simulink model "gm_hybrid_lht"  (R2019b)
settings: Solver=FixedStepDiscrete  StartTime=0.0  StopTime=inf  FixedStep=1/120e6  RelTol=1e-3
undefined symbols (not defined in the file or in its folder): bt, height, nTheta, width
libraries: hdlsllib x672, simulink x614, hdlmdlgenlib x7, dspsrcs4 x1
(part 10 of 18)

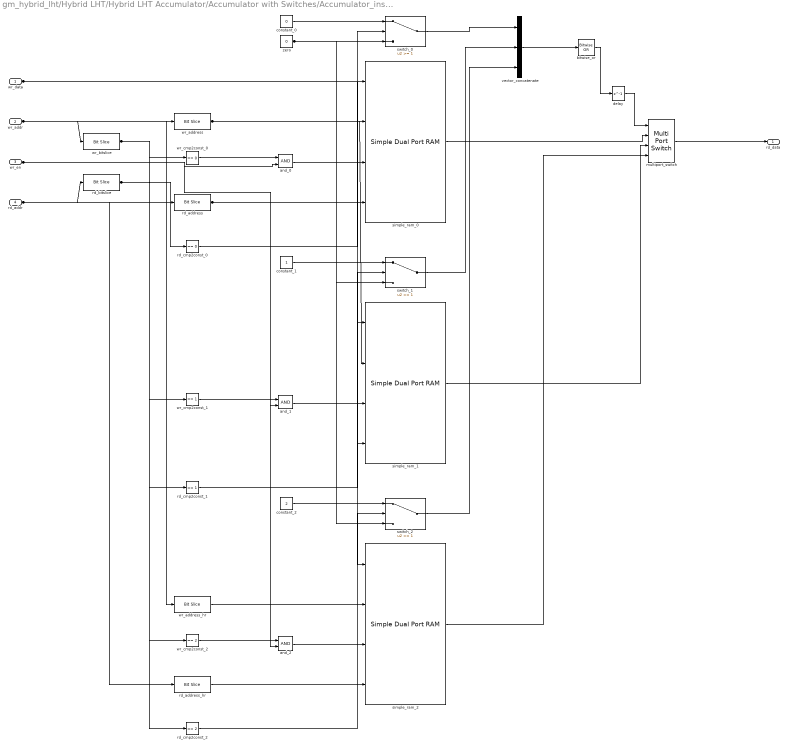
== system gm_hybrid_lht/Hybrid LHT/Hybrid LHT Accumulator/Accumulator with Switches/Accumulator_instance11/Block RAM/Simple Dual Port RAM Generator ==
  wr_data : Inport  OutDataTypeStr=fixdt(0, 36, 0)  PortDimensions=1  SampleTime=8.33333333333333e-09
  wr_addr : Inport  Port=2  OutDataTypeStr=fixdt(0, 12, 0)  PortDimensions=1  SampleTime=8.33333333333333e-09
  wr_en : Inport  Port=3  OutDataTypeStr=boolean  PortDimensions=1  SampleTime=8.33333333333333e-09
  rd_addr : Inport  Port=4  OutDataTypeStr=fixdt(0, 12, 0)  PortDimensions=1  SampleTime=8.33333333333333e-09
  and_0 : Logic  AllPortsSameDT=off  OutDataTypeStr=boolean
  and_1 : Logic  AllPortsSameDT=off  OutDataTypeStr=boolean
  and_2 : Logic  AllPortsSameDT=off  OutDataTypeStr=boolean
  bitwise_or : simulink/Logic and Bit Operations/Bitwise Operator  logicop=OR  UseBitMask=off  BitMask=bin2dec('11011001')  BitMaskRealWorld=Stored Integer
  constant_0 : Constant  Value=0  OutDataTypeStr=fixdt(0, 3, 0)  SampleTime=-1
  constant_1 : Constant  OutDataTypeStr=fixdt(0, 3, 0)  SampleTime=-1
  constant_2 : Constant  Value=2  OutDataTypeStr=fixdt(0, 3, 0)  SampleTime=-1
  delay : Delay  DelayLength=1
  multiport_switch : MultiPortSwitch  DataPortOrder=Zero-based contiguous  zeroidx=on
  rd_address : hdlsllib/Logic and Bit Operations/Bit Slice  lidx=9  ridx=0
      settings: SourceProductName=Simulink  SourceProductBaseCode=SL
  rd_address_hr : hdlsllib/Logic and Bit Operations/Bit Slice  lidx=8  ridx=0
      settings: SourceProductName=Simulink  SourceProductBaseCode=SL
  rd_bitslice : hdlsllib/Logic and Bit Operations/Bit Slice  lidx=11  ridx=10
      settings: SourceProductName=Simulink  SourceProductBaseCode=SL
  rd_cmp2const_0 : simulink/Logic and Bit Operations/Compare To Constant  relop===  const=0  OutDataTypeStr=boolean
  rd_cmp2const_1 : simulink/Logic and Bit Operations/Compare To Constant  relop===  const=1  OutDataTypeStr=boolean
  rd_cmp2const_2 : simulink/Logic and Bit Operations/Compare To Constant  relop===  const=2  OutDataTypeStr=boolean
  simple_ram_0 : hdlsllib/HDL RAMs/Simple Dual Port RAM  ram_size=10
      settings: SourceProductName=Simulink  SourceProductBaseCode=SL
  simple_ram_1 : hdlsllib/HDL RAMs/Simple Dual Port RAM  ram_size=10
      settings: SourceProductName=Simulink  SourceProductBaseCode=SL
  simple_ram_2 : hdlsllib/HDL RAMs/Simple Dual Port RAM  ram_size=9
      settings: SourceProductName=Simulink  SourceProductBaseCode=SL
  switch_0 : Switch  Threshold=1
  switch_1 : Switch  Threshold=1
  switch_2 : Switch  Threshold=1
  vector_concatenate : Concatenate  NumInputs=3
  wr_address : hdlsllib/Logic and Bit Operations/Bit Slice  lidx=9  ridx=0
      settings: SourceProductName=Simulink  SourceProductBaseCode=SL
  wr_address_hr : hdlsllib/Logic and Bit Operations/Bit Slice  lidx=8  ridx=0
      settings: SourceProductName=Simulink  SourceProductBaseCode=SL
  wr_bitslice : hdlsllib/Logic and Bit Operations/Bit Slice  lidx=11  ridx=10
      settings: SourceProductName=Simulink  SourceProductBaseCode=SL
  wr_cmp2const_0 : simulink/Logic and Bit Operations/Compare To Constant  relop===  const=0  OutDataTypeStr=boolean
  wr_cmp2const_1 : simulink/Logic and Bit Operations/Compare To Constant  relop===  const=1  OutDataTypeStr=boolean
  wr_cmp2const_2 : simulink/Logic and Bit Operations/Compare To Constant  relop===  const=2  OutDataTypeStr=boolean
  zero : Constant  Value=0  OutDataTypeStr=fixdt(0, 3, 0)  SampleTime=-1
  rd_data : Outport
  wires:
  rd_addr/1 -> rd_bitslice/1, rd_address_hr/1, rd_address/1
  wr_en/1 -> and_2/2, and_1/2, and_0/2
  wr_addr/1 -> wr_bitslice/1, wr_address_hr/1, wr_address/1
  wr_data/1 -> simple_ram_0/1, simple_ram_1/1, simple_ram_2/1
  and_0/1 -> simple_ram_0/3
  and_1/1 -> simple_ram_1/3
  and_2/1 -> simple_ram_2/3
  bitwise_or/1 -> delay/1
  constant_0/1 -> switch_0/1
  constant_1/1 -> switch_1/1
  constant_2/1 -> switch_2/1
  delay/1 -> multiport_switch/1
  multiport_switch/1 -> rd_data/1
  rd_address/1 -> simple_ram_0/4, simple_ram_1/4
  rd_address_hr/1 -> simple_ram_2/4
  rd_bitslice/1 -> rd_cmp2const_2/1, rd_cmp2const_1/1, rd_cmp2const_0/1
  rd_cmp2const_0/1 -> switch_0/2
  rd_cmp2const_1/1 -> switch_1/2
  rd_cmp2const_2/1 -> switch_2/2
  simple_ram_0/1 -> multiport_switch/2
  simple_ram_1/1 -> multiport_switch/3
  simple_ram_2/1 -> multiport_switch/4
  switch_0/1 -> vector_concatenate/1
  switch_1/1 -> vector_concatenate/2
  switch_2/1 -> vector_concatenate/3
  vector_concatenate/1 -> bitwise_or/1
  wr_address/1 -> simple_ram_0/2, simple_ram_1/2
  wr_address_hr/1 -> simple_ram_2/2
  wr_bitslice/1 -> wr_cmp2const_2/1, wr_cmp2const_1/1, wr_cmp2const_0/1
  wr_cmp2const_0/1 -> and_0/1
  wr_cmp2const_1/1 -> and_1/1
  wr_cmp2const_2/1 -> and_2/1
  zero/1 -> switch_2/3, switch_1/3, switch_0/3

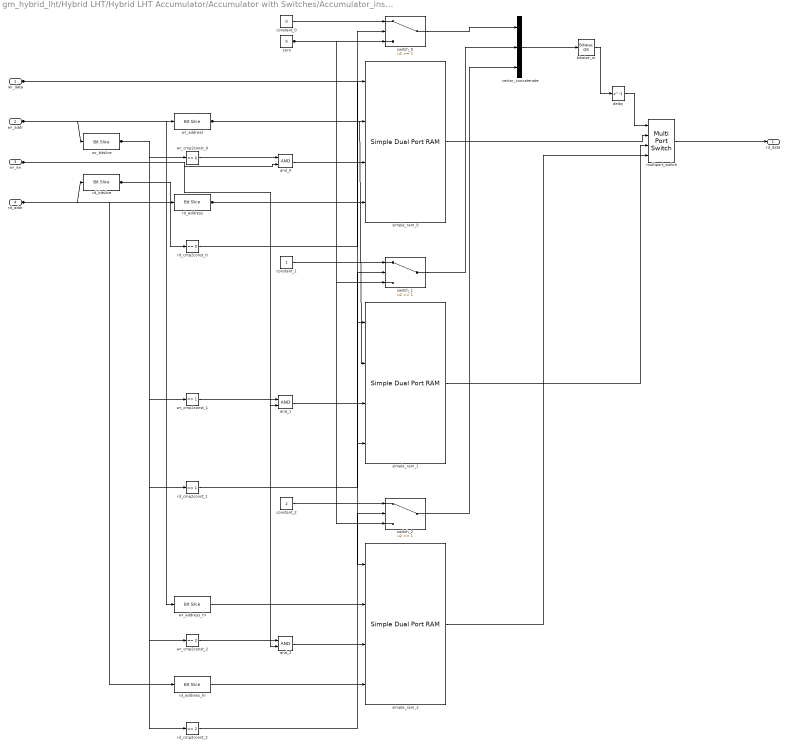
== system gm_hybrid_lht/Hybrid LHT/Hybrid LHT Accumulator/Accumulator with Switches/Accumulator_instance12/Block RAM/Simple Dual Port RAM Generator ==
  wr_data : Inport  OutDataTypeStr=fixdt(0, 36, 0)  PortDimensions=1  SampleTime=8.33333333333333e-09
  wr_addr : Inport  Port=2  OutDataTypeStr=fixdt(0, 12, 0)  PortDimensions=1  SampleTime=8.33333333333333e-09
  wr_en : Inport  Port=3  OutDataTypeStr=boolean  PortDimensions=1  SampleTime=8.33333333333333e-09
  rd_addr : Inport  Port=4  OutDataTypeStr=fixdt(0, 12, 0)  PortDimensions=1  SampleTime=8.33333333333333e-09
  and_0 : Logic  AllPortsSameDT=off  OutDataTypeStr=boolean
  and_1 : Logic  AllPortsSameDT=off  OutDataTypeStr=boolean
  and_2 : Logic  AllPortsSameDT=off  OutDataTypeStr=boolean
  bitwise_or : simulink/Logic and Bit Operations/Bitwise Operator  logicop=OR  UseBitMask=off  BitMask=bin2dec('11011001')  BitMaskRealWorld=Stored Integer
  constant_0 : Constant  Value=0  OutDataTypeStr=fixdt(0, 3, 0)  SampleTime=-1
  constant_1 : Constant  OutDataTypeStr=fixdt(0, 3, 0)  SampleTime=-1
  constant_2 : Constant  Value=2  OutDataTypeStr=fixdt(0, 3, 0)  SampleTime=-1
  delay : Delay  DelayLength=1
  multiport_switch : MultiPortSwitch  DataPortOrder=Zero-based contiguous  zeroidx=on
  rd_address : hdlsllib/Logic and Bit Operations/Bit Slice  lidx=9  ridx=0
      settings: SourceProductName=Simulink  SourceProductBaseCode=SL
  rd_address_hr : hdlsllib/Logic and Bit Operations/Bit Slice  lidx=8  ridx=0
      settings: SourceProductName=Simulink  SourceProductBaseCode=SL
  rd_bitslice : hdlsllib/Logic and Bit Operations/Bit Slice  lidx=11  ridx=10
      settings: SourceProductName=Simulink  SourceProductBaseCode=SL
  rd_cmp2const_0 : simulink/Logic and Bit Operations/Compare To Constant  relop===  const=0  OutDataTypeStr=boolean
  rd_cmp2const_1 : simulink/Logic and Bit Operations/Compare To Constant  relop===  const=1  OutDataTypeStr=boolean
  rd_cmp2const_2 : simulink/Logic and Bit Operations/Compare To Constant  relop===  const=2  OutDataTypeStr=boolean
  simple_ram_0 : hdlsllib/HDL RAMs/Simple Dual Port RAM  ram_size=10
      settings: SourceProductName=Simulink  SourceProductBaseCode=SL
  simple_ram_1 : hdlsllib/HDL RAMs/Simple Dual Port RAM  ram_size=10
      settings: SourceProductName=Simulink  SourceProductBaseCode=SL
  simple_ram_2 : hdlsllib/HDL RAMs/Simple Dual Port RAM  ram_size=9
      settings: SourceProductName=Simulink  SourceProductBaseCode=SL
  switch_0 : Switch  Threshold=1
  switch_1 : Switch  Threshold=1
  switch_2 : Switch  Threshold=1
  vector_concatenate : Concatenate  NumInputs=3
  wr_address : hdlsllib/Logic and Bit Operations/Bit Slice  lidx=9  ridx=0
      settings: SourceProductName=Simulink  SourceProductBaseCode=SL
  wr_address_hr : hdlsllib/Logic and Bit Operations/Bit Slice  lidx=8  ridx=0
      settings: SourceProductName=Simulink  SourceProductBaseCode=SL
  wr_bitslice : hdlsllib/Logic and Bit Operations/Bit Slice  lidx=11  ridx=10
      settings: SourceProductName=Simulink  SourceProductBaseCode=SL
  wr_cmp2const_0 : simulink/Logic and Bit Operations/Compare To Constant  relop===  const=0  OutDataTypeStr=boolean
  wr_cmp2const_1 : simulink/Logic and Bit Operations/Compare To Constant  relop===  const=1  OutDataTypeStr=boolean
  wr_cmp2const_2 : simulink/Logic and Bit Operations/Compare To Constant  relop===  const=2  OutDataTypeStr=boolean
  zero : Constant  Value=0  OutDataTypeStr=fixdt(0, 3, 0)  SampleTime=-1
  rd_data : Outport
  wires:
  rd_addr/1 -> rd_bitslice/1, rd_address_hr/1, rd_address/1
  wr_en/1 -> and_2/2, and_1/2, and_0/2
  wr_addr/1 -> wr_bitslice/1, wr_address_hr/1, wr_address/1
  wr_data/1 -> simple_ram_0/1, simple_ram_1/1, simple_ram_2/1
  and_0/1 -> simple_ram_0/3
  and_1/1 -> simple_ram_1/3
  and_2/1 -> simple_ram_2/3
  bitwise_or/1 -> delay/1
  constant_0/1 -> switch_0/1
  constant_1/1 -> switch_1/1
  constant_2/1 -> switch_2/1
  delay/1 -> multiport_switch/1
  multiport_switch/1 -> rd_data/1
  rd_address/1 -> simple_ram_0/4, simple_ram_1/4
  rd_address_hr/1 -> simple_ram_2/4
  rd_bitslice/1 -> rd_cmp2const_2/1, rd_cmp2const_1/1, rd_cmp2const_0/1
  rd_cmp2const_0/1 -> switch_0/2
  rd_cmp2const_1/1 -> switch_1/2
  rd_cmp2const_2/1 -> switch_2/2
  simple_ram_0/1 -> multiport_switch/2
  simple_ram_1/1 -> multiport_switch/3
  simple_ram_2/1 -> multiport_switch/4
  switch_0/1 -> vector_concatenate/1
  switch_1/1 -> vector_concatenate/2
  switch_2/1 -> vector_concatenate/3
  vector_concatenate/1 -> bitwise_or/1
  wr_address/1 -> simple_ram_0/2, simple_ram_1/2
  wr_address_hr/1 -> simple_ram_2/2
  wr_bitslice/1 -> wr_cmp2const_2/1, wr_cmp2const_1/1, wr_cmp2const_0/1
  wr_cmp2const_0/1 -> and_0/1
  wr_cmp2const_1/1 -> and_1/1
  wr_cmp2const_2/1 -> and_2/1
  zero/1 -> switch_2/3, switch_1/3, switch_0/3

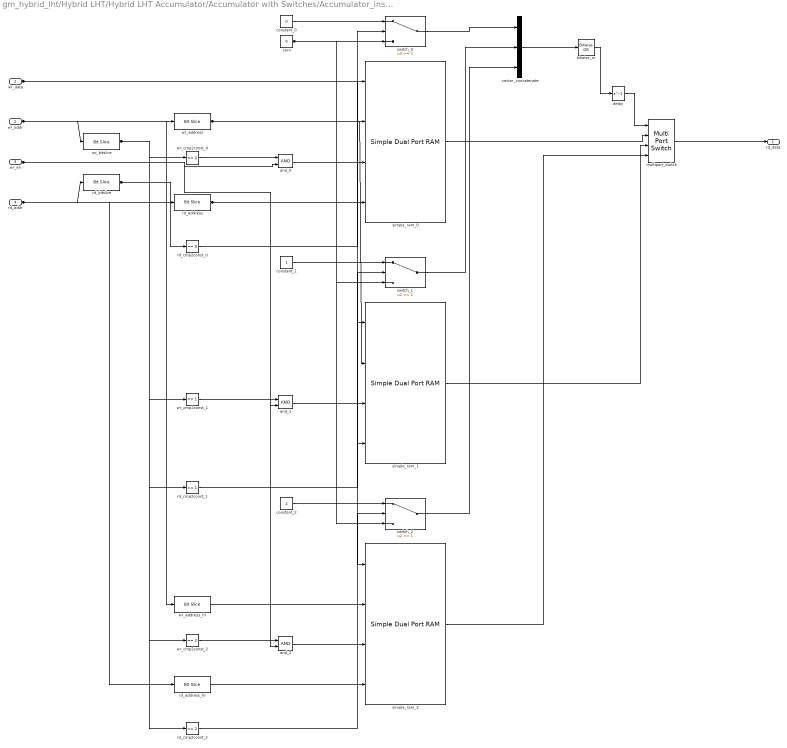
== system gm_hybrid_lht/Hybrid LHT/Hybrid LHT Accumulator/Accumulator with Switches/Accumulator_instance13/Block RAM/Simple Dual Port RAM Generator ==
  wr_data : Inport  OutDataTypeStr=fixdt(0, 36, 0)  PortDimensions=1  SampleTime=8.33333333333333e-09
  wr_addr : Inport  Port=2  OutDataTypeStr=fixdt(0, 12, 0)  PortDimensions=1  SampleTime=8.33333333333333e-09
  wr_en : Inport  Port=3  OutDataTypeStr=boolean  PortDimensions=1  SampleTime=8.33333333333333e-09
  rd_addr : Inport  Port=4  OutDataTypeStr=fixdt(0, 12, 0)  PortDimensions=1  SampleTime=8.33333333333333e-09
  and_0 : Logic  AllPortsSameDT=off  OutDataTypeStr=boolean
  and_1 : Logic  AllPortsSameDT=off  OutDataTypeStr=boolean
  and_2 : Logic  AllPortsSameDT=off  OutDataTypeStr=boolean
  bitwise_or : simulink/Logic and Bit Operations/Bitwise Operator  logicop=OR  UseBitMask=off  BitMask=bin2dec('11011001')  BitMaskRealWorld=Stored Integer
  constant_0 : Constant  Value=0  OutDataTypeStr=fixdt(0, 3, 0)  SampleTime=-1
  constant_1 : Constant  OutDataTypeStr=fixdt(0, 3, 0)  SampleTime=-1
  constant_2 : Constant  Value=2  OutDataTypeStr=fixdt(0, 3, 0)  SampleTime=-1
  delay : Delay  DelayLength=1
  multiport_switch : MultiPortSwitch  DataPortOrder=Zero-based contiguous  zeroidx=on
  rd_address : hdlsllib/Logic and Bit Operations/Bit Slice  lidx=9  ridx=0
      settings: SourceProductName=Simulink  SourceProductBaseCode=SL
  rd_address_hr : hdlsllib/Logic and Bit Operations/Bit Slice  lidx=8  ridx=0
      settings: SourceProductName=Simulink  SourceProductBaseCode=SL
  rd_bitslice : hdlsllib/Logic and Bit Operations/Bit Slice  lidx=11  ridx=10
      settings: SourceProductName=Simulink  SourceProductBaseCode=SL
  rd_cmp2const_0 : simulink/Logic and Bit Operations/Compare To Constant  relop===  const=0  OutDataTypeStr=boolean
  rd_cmp2const_1 : simulink/Logic and Bit Operations/Compare To Constant  relop===  const=1  OutDataTypeStr=boolean
  rd_cmp2const_2 : simulink/Logic and Bit Operations/Compare To Constant  relop===  const=2  OutDataTypeStr=boolean
  simple_ram_0 : hdlsllib/HDL RAMs/Simple Dual Port RAM  ram_size=10
      settings: SourceProductName=Simulink  SourceProductBaseCode=SL
  simple_ram_1 : hdlsllib/HDL RAMs/Simple Dual Port RAM  ram_size=10
      settings: SourceProductName=Simulink  SourceProductBaseCode=SL
  simple_ram_2 : hdlsllib/HDL RAMs/Simple Dual Port RAM  ram_size=9
      settings: SourceProductName=Simulink  SourceProductBaseCode=SL
  switch_0 : Switch  Threshold=1
  switch_1 : Switch  Threshold=1
  switch_2 : Switch  Threshold=1
  vector_concatenate : Concatenate  NumInputs=3
  wr_address : hdlsllib/Logic and Bit Operations/Bit Slice  lidx=9  ridx=0
      settings: SourceProductName=Simulink  SourceProductBaseCode=SL
  wr_address_hr : hdlsllib/Logic and Bit Operations/Bit Slice  lidx=8  ridx=0
      settings: SourceProductName=Simulink  SourceProductBaseCode=SL
  wr_bitslice : hdlsllib/Logic and Bit Operations/Bit Slice  lidx=11  ridx=10
      settings: SourceProductName=Simulink  SourceProductBaseCode=SL
  wr_cmp2const_0 : simulink/Logic and Bit Operations/Compare To Constant  relop===  const=0  OutDataTypeStr=boolean
  wr_cmp2const_1 : simulink/Logic and Bit Operations/Compare To Constant  relop===  const=1  OutDataTypeStr=boolean
  wr_cmp2const_2 : simulink/Logic and Bit Operations/Compare To Constant  relop===  const=2  OutDataTypeStr=boolean
  zero : Constant  Value=0  OutDataTypeStr=fixdt(0, 3, 0)  SampleTime=-1
  rd_data : Outport
  wires:
  rd_addr/1 -> rd_bitslice/1, rd_address_hr/1, rd_address/1
  wr_en/1 -> and_2/2, and_1/2, and_0/2
  wr_addr/1 -> wr_bitslice/1, wr_address_hr/1, wr_address/1
  wr_data/1 -> simple_ram_0/1, simple_ram_1/1, simple_ram_2/1
  and_0/1 -> simple_ram_0/3
  and_1/1 -> simple_ram_1/3
  and_2/1 -> simple_ram_2/3
  bitwise_or/1 -> delay/1
  constant_0/1 -> switch_0/1
  constant_1/1 -> switch_1/1
  constant_2/1 -> switch_2/1
  delay/1 -> multiport_switch/1
  multiport_switch/1 -> rd_data/1
  rd_address/1 -> simple_ram_0/4, simple_ram_1/4
  rd_address_hr/1 -> simple_ram_2/4
  rd_bitslice/1 -> rd_cmp2const_2/1, rd_cmp2const_1/1, rd_cmp2const_0/1
  rd_cmp2const_0/1 -> switch_0/2
  rd_cmp2const_1/1 -> switch_1/2
  rd_cmp2const_2/1 -> switch_2/2
  simple_ram_0/1 -> multiport_switch/2
  simple_ram_1/1 -> multiport_switch/3
  simple_ram_2/1 -> multiport_switch/4
  switch_0/1 -> vector_concatenate/1
  switch_1/1 -> vector_concatenate/2
  switch_2/1 -> vector_concatenate/3
  vector_concatenate/1 -> bitwise_or/1
  wr_address/1 -> simple_ram_0/2, simple_ram_1/2
  wr_address_hr/1 -> simple_ram_2/2
  wr_bitslice/1 -> wr_cmp2const_2/1, wr_cmp2const_1/1, wr_cmp2const_0/1
  wr_cmp2const_0/1 -> and_0/1
  wr_cmp2const_1/1 -> and_1/1
  wr_cmp2const_2/1 -> and_2/1
  zero/1 -> switch_2/3, switch_1/3, switch_0/3

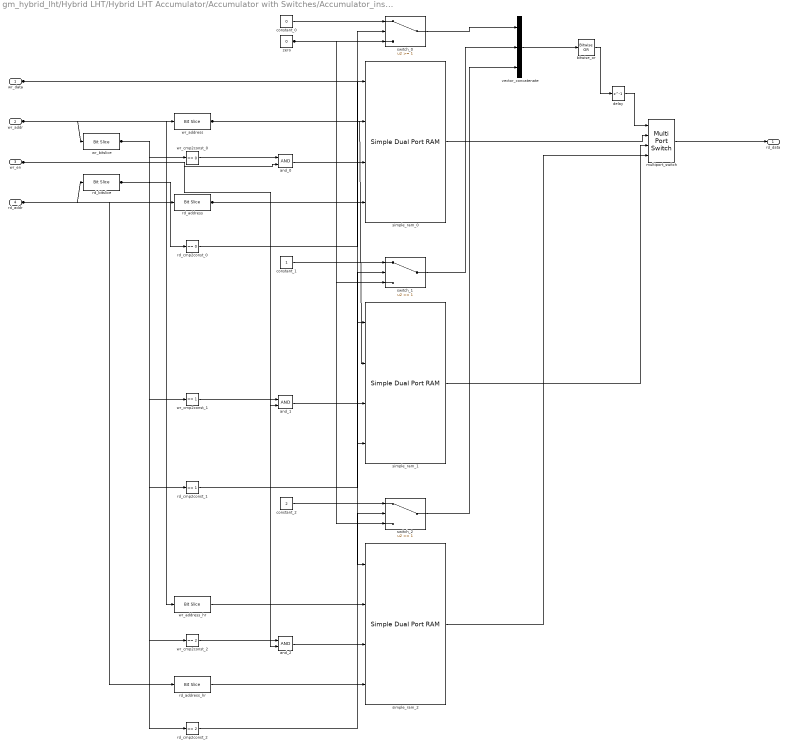
== system gm_hybrid_lht/Hybrid LHT/Hybrid LHT Accumulator/Accumulator with Switches/Accumulator_instance14/Block RAM/Simple Dual Port RAM Generator ==
  wr_data : Inport  OutDataTypeStr=fixdt(0, 36, 0)  PortDimensions=1  SampleTime=8.33333333333333e-09
  wr_addr : Inport  Port=2  OutDataTypeStr=fixdt(0, 12, 0)  PortDimensions=1  SampleTime=8.33333333333333e-09
  wr_en : Inport  Port=3  OutDataTypeStr=boolean  PortDimensions=1  SampleTime=8.33333333333333e-09
  rd_addr : Inport  Port=4  OutDataTypeStr=fixdt(0, 12, 0)  PortDimensions=1  SampleTime=8.33333333333333e-09
  and_0 : Logic  AllPortsSameDT=off  OutDataTypeStr=boolean
  and_1 : Logic  AllPortsSameDT=off  OutDataTypeStr=boolean
  and_2 : Logic  AllPortsSameDT=off  OutDataTypeStr=boolean
  bitwise_or : simulink/Logic and Bit Operations/Bitwise Operator  logicop=OR  UseBitMask=off  BitMask=bin2dec('11011001')  BitMaskRealWorld=Stored Integer
  constant_0 : Constant  Value=0  OutDataTypeStr=fixdt(0, 3, 0)  SampleTime=-1
  constant_1 : Constant  OutDataTypeStr=fixdt(0, 3, 0)  SampleTime=-1
  constant_2 : Constant  Value=2  OutDataTypeStr=fixdt(0, 3, 0)  SampleTime=-1
  delay : Delay  DelayLength=1
  multiport_switch : MultiPortSwitch  DataPortOrder=Zero-based contiguous  zeroidx=on
  rd_address : hdlsllib/Logic and Bit Operations/Bit Slice  lidx=9  ridx=0
      settings: SourceProductName=Simulink  SourceProductBaseCode=SL
  rd_address_hr : hdlsllib/Logic and Bit Operations/Bit Slice  lidx=8  ridx=0
      settings: SourceProductName=Simulink  SourceProductBaseCode=SL
  rd_bitslice : hdlsllib/Logic and Bit Operations/Bit Slice  lidx=11  ridx=10
      settings: SourceProductName=Simulink  SourceProductBaseCode=SL
  rd_cmp2const_0 : simulink/Logic and Bit Operations/Compare To Constant  relop===  const=0  OutDataTypeStr=boolean
  rd_cmp2const_1 : simulink/Logic and Bit Operations/Compare To Constant  relop===  const=1  OutDataTypeStr=boolean
  rd_cmp2const_2 : simulink/Logic and Bit Operations/Compare To Constant  relop===  const=2  OutDataTypeStr=boolean
  simple_ram_0 : hdlsllib/HDL RAMs/Simple Dual Port RAM  ram_size=10
      settings: SourceProductName=Simulink  SourceProductBaseCode=SL
  simple_ram_1 : hdlsllib/HDL RAMs/Simple Dual Port RAM  ram_size=10
      settings: SourceProductName=Simulink  SourceProductBaseCode=SL
  simple_ram_2 : hdlsllib/HDL RAMs/Simple Dual Port RAM  ram_size=9
      settings: SourceProductName=Simulink  SourceProductBaseCode=SL
  switch_0 : Switch  Threshold=1
  switch_1 : Switch  Threshold=1
  switch_2 : Switch  Threshold=1
  vector_concatenate : Concatenate  NumInputs=3
  wr_address : hdlsllib/Logic and Bit Operations/Bit Slice  lidx=9  ridx=0
      settings: SourceProductName=Simulink  SourceProductBaseCode=SL
  wr_address_hr : hdlsllib/Logic and Bit Operations/Bit Slice  lidx=8  ridx=0
      settings: SourceProductName=Simulink  SourceProductBaseCode=SL
  wr_bitslice : hdlsllib/Logic and Bit Operations/Bit Slice  lidx=11  ridx=10
      settings: SourceProductName=Simulink  SourceProductBaseCode=SL
  wr_cmp2const_0 : simulink/Logic and Bit Operations/Compare To Constant  relop===  const=0  OutDataTypeStr=boolean
  wr_cmp2const_1 : simulink/Logic and Bit Operations/Compare To Constant  relop===  const=1  OutDataTypeStr=boolean
  wr_cmp2const_2 : simulink/Logic and Bit Operations/Compare To Constant  relop===  const=2  OutDataTypeStr=boolean
  zero : Constant  Value=0  OutDataTypeStr=fixdt(0, 3, 0)  SampleTime=-1
  rd_data : Outport
  wires:
  rd_addr/1 -> rd_bitslice/1, rd_address_hr/1, rd_address/1
  wr_en/1 -> and_2/2, and_1/2, and_0/2
  wr_addr/1 -> wr_bitslice/1, wr_address_hr/1, wr_address/1
  wr_data/1 -> simple_ram_0/1, simple_ram_1/1, simple_ram_2/1
  and_0/1 -> simple_ram_0/3
  and_1/1 -> simple_ram_1/3
  and_2/1 -> simple_ram_2/3
  bitwise_or/1 -> delay/1
  constant_0/1 -> switch_0/1
  constant_1/1 -> switch_1/1
  constant_2/1 -> switch_2/1
  delay/1 -> multiport_switch/1
  multiport_switch/1 -> rd_data/1
  rd_address/1 -> simple_ram_0/4, simple_ram_1/4
  rd_address_hr/1 -> simple_ram_2/4
  rd_bitslice/1 -> rd_cmp2const_2/1, rd_cmp2const_1/1, rd_cmp2const_0/1
  rd_cmp2const_0/1 -> switch_0/2
  rd_cmp2const_1/1 -> switch_1/2
  rd_cmp2const_2/1 -> switch_2/2
  simple_ram_0/1 -> multiport_switch/2
  simple_ram_1/1 -> multiport_switch/3
  simple_ram_2/1 -> multiport_switch/4
  switch_0/1 -> vector_concatenate/1
  switch_1/1 -> vector_concatenate/2
  switch_2/1 -> vector_concatenate/3
  vector_concatenate/1 -> bitwise_or/1
  wr_address/1 -> simple_ram_0/2, simple_ram_1/2
  wr_address_hr/1 -> simple_ram_2/2
  wr_bitslice/1 -> wr_cmp2const_2/1, wr_cmp2const_1/1, wr_cmp2const_0/1
  wr_cmp2const_0/1 -> and_0/1
  wr_cmp2const_1/1 -> and_1/1
  wr_cmp2const_2/1 -> and_2/1
  zero/1 -> switch_2/3, switch_1/3, switch_0/3

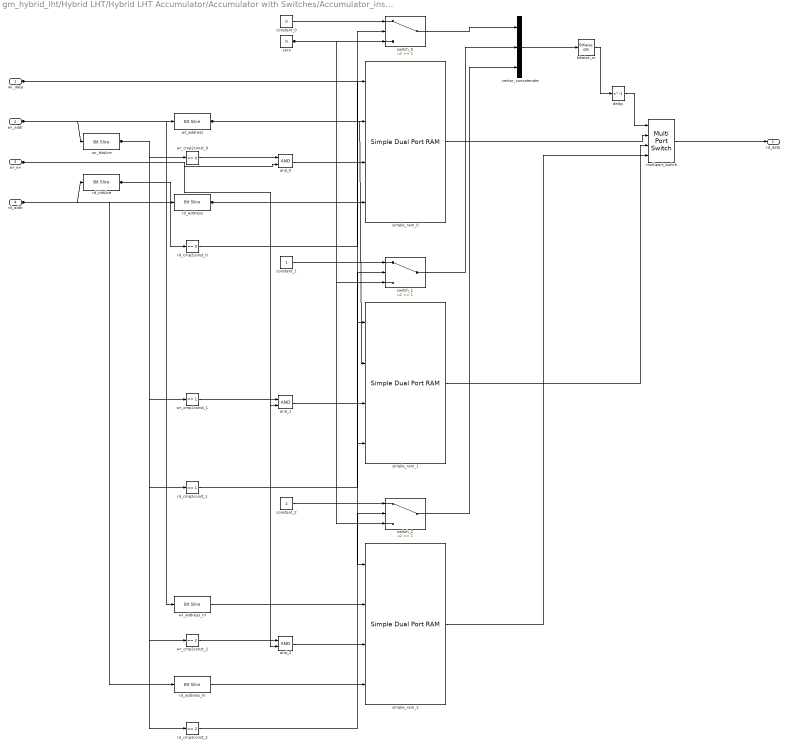
== system gm_hybrid_lht/Hybrid LHT/Hybrid LHT Accumulator/Accumulator with Switches/Accumulator_instance15/Block RAM/Simple Dual Port RAM Generator ==
  wr_data : Inport  OutDataTypeStr=fixdt(0, 36, 0)  PortDimensions=1  SampleTime=8.33333333333333e-09
  wr_addr : Inport  Port=2  OutDataTypeStr=fixdt(0, 12, 0)  PortDimensions=1  SampleTime=8.33333333333333e-09
  wr_en : Inport  Port=3  OutDataTypeStr=boolean  PortDimensions=1  SampleTime=8.33333333333333e-09
  rd_addr : Inport  Port=4  OutDataTypeStr=fixdt(0, 12, 0)  PortDimensions=1  SampleTime=8.33333333333333e-09
  and_0 : Logic  AllPortsSameDT=off  OutDataTypeStr=boolean
  and_1 : Logic  AllPortsSameDT=off  OutDataTypeStr=boolean
  and_2 : Logic  AllPortsSameDT=off  OutDataTypeStr=boolean
  bitwise_or : simulink/Logic and Bit Operations/Bitwise Operator  logicop=OR  UseBitMask=off  BitMask=bin2dec('11011001')  BitMaskRealWorld=Stored Integer
  constant_0 : Constant  Value=0  OutDataTypeStr=fixdt(0, 3, 0)  SampleTime=-1
  constant_1 : Constant  OutDataTypeStr=fixdt(0, 3, 0)  SampleTime=-1
  constant_2 : Constant  Value=2  OutDataTypeStr=fixdt(0, 3, 0)  SampleTime=-1
  delay : Delay  DelayLength=1
  multiport_switch : MultiPortSwitch  DataPortOrder=Zero-based contiguous  zeroidx=on
  rd_address : hdlsllib/Logic and Bit Operations/Bit Slice  lidx=9  ridx=0
      settings: SourceProductName=Simulink  SourceProductBaseCode=SL
  rd_address_hr : hdlsllib/Logic and Bit Operations/Bit Slice  lidx=8  ridx=0
      settings: SourceProductName=Simulink  SourceProductBaseCode=SL
  rd_bitslice : hdlsllib/Logic and Bit Operations/Bit Slice  lidx=11  ridx=10
      settings: SourceProductName=Simulink  SourceProductBaseCode=SL
  rd_cmp2const_0 : simulink/Logic and Bit Operations/Compare To Constant  relop===  const=0  OutDataTypeStr=boolean
  rd_cmp2const_1 : simulink/Logic and Bit Operations/Compare To Constant  relop===  const=1  OutDataTypeStr=boolean
  rd_cmp2const_2 : simulink/Logic and Bit Operations/Compare To Constant  relop===  const=2  OutDataTypeStr=boolean
  simple_ram_0 : hdlsllib/HDL RAMs/Simple Dual Port RAM  ram_size=10
      settings: SourceProductName=Simulink  SourceProductBaseCode=SL
  simple_ram_1 : hdlsllib/HDL RAMs/Simple Dual Port RAM  ram_size=10
      settings: SourceProductName=Simulink  SourceProductBaseCode=SL
  simple_ram_2 : hdlsllib/HDL RAMs/Simple Dual Port RAM  ram_size=9
      settings: SourceProductName=Simulink  SourceProductBaseCode=SL
  switch_0 : Switch  Threshold=1
  switch_1 : Switch  Threshold=1
  switch_2 : Switch  Threshold=1
  vector_concatenate : Concatenate  NumInputs=3
  wr_address : hdlsllib/Logic and Bit Operations/Bit Slice  lidx=9  ridx=0
      settings: SourceProductName=Simulink  SourceProductBaseCode=SL
  wr_address_hr : hdlsllib/Logic and Bit Operations/Bit Slice  lidx=8  ridx=0
      settings: SourceProductName=Simulink  SourceProductBaseCode=SL
  wr_bitslice : hdlsllib/Logic and Bit Operations/Bit Slice  lidx=11  ridx=10
      settings: SourceProductName=Simulink  SourceProductBaseCode=SL
  wr_cmp2const_0 : simulink/Logic and Bit Operations/Compare To Constant  relop===  const=0  OutDataTypeStr=boolean
  wr_cmp2const_1 : simulink/Logic and Bit Operations/Compare To Constant  relop===  const=1  OutDataTypeStr=boolean
  wr_cmp2const_2 : simulink/Logic and Bit Operations/Compare To Constant  relop===  const=2  OutDataTypeStr=boolean
  zero : Constant  Value=0  OutDataTypeStr=fixdt(0, 3, 0)  SampleTime=-1
  rd_data : Outport
  wires:
  rd_addr/1 -> rd_bitslice/1, rd_address_hr/1, rd_address/1
  wr_en/1 -> and_2/2, and_1/2, and_0/2
  wr_addr/1 -> wr_bitslice/1, wr_address_hr/1, wr_address/1
  wr_data/1 -> simple_ram_0/1, simple_ram_1/1, simple_ram_2/1
  and_0/1 -> simple_ram_0/3
  and_1/1 -> simple_ram_1/3
  and_2/1 -> simple_ram_2/3
  bitwise_or/1 -> delay/1
  constant_0/1 -> switch_0/1
  constant_1/1 -> switch_1/1
  constant_2/1 -> switch_2/1
  delay/1 -> multiport_switch/1
  multiport_switch/1 -> rd_data/1
  rd_address/1 -> simple_ram_0/4, simple_ram_1/4
  rd_address_hr/1 -> simple_ram_2/4
  rd_bitslice/1 -> rd_cmp2const_2/1, rd_cmp2const_1/1, rd_cmp2const_0/1
  rd_cmp2const_0/1 -> switch_0/2
  rd_cmp2const_1/1 -> switch_1/2
  rd_cmp2const_2/1 -> switch_2/2
  simple_ram_0/1 -> multiport_switch/2
  simple_ram_1/1 -> multiport_switch/3
  simple_ram_2/1 -> multiport_switch/4
  switch_0/1 -> vector_concatenate/1
  switch_1/1 -> vector_concatenate/2
  switch_2/1 -> vector_concatenate/3
  vector_concatenate/1 -> bitwise_or/1
  wr_address/1 -> simple_ram_0/2, simple_ram_1/2
  wr_address_hr/1 -> simple_ram_2/2
  wr_bitslice/1 -> wr_cmp2const_2/1, wr_cmp2const_1/1, wr_cmp2const_0/1
  wr_cmp2const_0/1 -> and_0/1
  wr_cmp2const_1/1 -> and_1/1
  wr_cmp2const_2/1 -> and_2/1
  zero/1 -> switch_2/3, switch_1/3, switch_0/3

== system gm_hybrid_lht/Hybrid LHT/Hybrid LHT Accumulator/Accumulator with Switches/Accumulator_instance16/Block RAM/Simple Dual Port RAM Generator ==
  wr_data : Inport  OutDataTypeStr=fixdt(0, 36, 0)  PortDimensions=1  SampleTime=8.33333333333333e-09
  wr_addr : Inport  Port=2  OutDataTypeStr=fixdt(0, 12, 0)  PortDimensions=1  SampleTime=8.33333333333333e-09
  wr_en : Inport  Port=3  OutDataTypeStr=boolean  PortDimensions=1  SampleTime=8.33333333333333e-09
  rd_addr : Inport  Port=4  OutDataTypeStr=fixdt(0, 12, 0)  PortDimensions=1  SampleTime=8.33333333333333e-09
  and_0 : Logic  AllPortsSameDT=off  OutDataTypeStr=boolean
  and_1 : Logic  AllPortsSameDT=off  OutDataTypeStr=boolean
  and_2 : Logic  AllPortsSameDT=off  OutDataTypeStr=boolean
  bitwise_or : simulink/Logic and Bit Operations/Bitwise Operator  logicop=OR  UseBitMask=off  BitMask=bin2dec('11011001')  BitMaskRealWorld=Stored Integer
  constant_0 : Constant  Value=0  OutDataTypeStr=fixdt(0, 3, 0)  SampleTime=-1
  constant_1 : Constant  OutDataTypeStr=fixdt(0, 3, 0)  SampleTime=-1
  constant_2 : Constant  Value=2  OutDataTypeStr=fixdt(0, 3, 0)  SampleTime=-1
  delay : Delay  DelayLength=1
  multiport_switch : MultiPortSwitch  DataPortOrder=Zero-based contiguous  zeroidx=on
  rd_address : hdlsllib/Logic and Bit Operations/Bit Slice  lidx=9  ridx=0
      settings: SourceProductName=Simulink  SourceProductBaseCode=SL
  rd_address_hr : hdlsllib/Logic and Bit Operations/Bit Slice  lidx=8  ridx=0
      settings: SourceProductName=Simulink  SourceProductBaseCode=SL
  rd_bitslice : hdlsllib/Logic and Bit Operations/Bit Slice  lidx=11  ridx=10
      settings: SourceProductName=Simulink  SourceProductBaseCode=SL
  rd_cmp2const_0 : simulink/Logic and Bit Operations/Compare To Constant  relop===  const=0  OutDataTypeStr=boolean
  rd_cmp2const_1 : simulink/Logic and Bit Operations/Compare To Constant  relop===  const=1  OutDataTypeStr=boolean
  rd_cmp2const_2 : simulink/Logic and Bit Operations/Compare To Constant  relop===  const=2  OutDataTypeStr=boolean
  simple_ram_0 : hdlsllib/HDL RAMs/Simple Dual Port RAM  ram_size=10
      settings: SourceProductName=Simulink  SourceProductBaseCode=SL
  simple_ram_1 : hdlsllib/HDL RAMs/Simple Dual Port RAM  ram_size=10
      settings: SourceProductName=Simulink  SourceProductBaseCode=SL
  simple_ram_2 : hdlsllib/HDL RAMs/Simple Dual Port RAM  ram_size=9
      settings: SourceProductName=Simulink  SourceProductBaseCode=SL
  switch_0 : Switch  Threshold=1
  switch_1 : Switch  Threshold=1
  switch_2 : Switch  Threshold=1
  vector_concatenate : Concatenate  NumInputs=3
  wr_address : hdlsllib/Logic and Bit Operations/Bit Slice  lidx=9  ridx=0
      settings: SourceProductName=Simulink  SourceProductBaseCode=SL
  wr_address_hr : hdlsllib/Logic and Bit Operations/Bit Slice  lidx=8  ridx=0
      settings: SourceProductName=Simulink  SourceProductBaseCode=SL
  wr_bitslice : hdlsllib/Logic and Bit Operations/Bit Slice  lidx=11  ridx=10
      settings: SourceProductName=Simulink  SourceProductBaseCode=SL
  wr_cmp2const_0 : simulink/Logic and Bit Operations/Compare To Constant  relop===  const=0  OutDataTypeStr=boolean
  wr_cmp2const_1 : simulink/Logic and Bit Operations/Compare To Constant  relop===  const=1  OutDataTypeStr=boolean
  wr_cmp2const_2 : simulink/Logic and Bit Operations/Compare To Constant  relop===  const=2  OutDataTypeStr=boolean
  zero : Constant  Value=0  OutDataTypeStr=fixdt(0, 3, 0)  SampleTime=-1
  rd_data : Outport
  wires:
  rd_addr/1 -> rd_bitslice/1, rd_address_hr/1, rd_address/1
  wr_en/1 -> and_2/2, and_1/2, and_0/2
  wr_addr/1 -> wr_bitslice/1, wr_address_hr/1, wr_address/1
  wr_data/1 -> simple_ram_0/1, simple_ram_1/1, simple_ram_2/1
  and_0/1 -> simple_ram_0/3
  and_1/1 -> simple_ram_1/3
  and_2/1 -> simple_ram_2/3
  bitwise_or/1 -> delay/1
  constant_0/1 -> switch_0/1
  constant_1/1 -> switch_1/1
  constant_2/1 -> switch_2/1
  delay/1 -> multiport_switch/1
  multiport_switch/1 -> rd_data/1
  rd_address/1 -> simple_ram_0/4, simple_ram_1/4
  rd_address_hr/1 -> simple_ram_2/4
  rd_bitslice/1 -> rd_cmp2const_2/1, rd_cmp2const_1/1, rd_cmp2const_0/1
  rd_cmp2const_0/1 -> switch_0/2
  rd_cmp2const_1/1 -> switch_1/2
  rd_cmp2const_2/1 -> switch_2/2
  simple_ram_0/1 -> multiport_switch/2
  simple_ram_1/1 -> multiport_switch/3
  simple_ram_2/1 -> multiport_switch/4
  switch_0/1 -> vector_concatenate/1
  switch_1/1 -> vector_concatenate/2
  switch_2/1 -> vector_concatenate/3
  vector_concatenate/1 -> bitwise_or/1
  wr_address/1 -> simple_ram_0/2, simple_ram_1/2
  wr_address_hr/1 -> simple_ram_2/2
  wr_bitslice/1 -> wr_cmp2const_2/1, wr_cmp2const_1/1, wr_cmp2const_0/1
  wr_cmp2const_0/1 -> and_0/1
  wr_cmp2const_1/1 -> and_1/1
  wr_cmp2const_2/1 -> and_2/1
  zero/1 -> switch_2/3, switch_1/3, switch_0/3

== system gm_hybrid_lht/Hybrid LHT/Hybrid LHT Accumulator/Accumulator with Switches/Accumulator_instance17/Block RAM/Simple Dual Port RAM Generator ==
  wr_data : Inport  OutDataTypeStr=fixdt(0, 36, 0)  PortDimensions=1  SampleTime=8.33333333333333e-09
  wr_addr : Inport  Port=2  OutDataTypeStr=fixdt(0, 12, 0)  PortDimensions=1  SampleTime=8.33333333333333e-09
  wr_en : Inport  Port=3  OutDataTypeStr=boolean  PortDimensions=1  SampleTime=8.33333333333333e-09
  rd_addr : Inport  Port=4  OutDataTypeStr=fixdt(0, 12, 0)  PortDimensions=1  SampleTime=8.33333333333333e-09
  and_0 : Logic  AllPortsSameDT=off  OutDataTypeStr=boolean
  and_1 : Logic  AllPortsSameDT=off  OutDataTypeStr=boolean
  and_2 : Logic  AllPortsSameDT=off  OutDataTypeStr=boolean
  bitwise_or : simulink/Logic and Bit Operations/Bitwise Operator  logicop=OR  UseBitMask=off  BitMask=bin2dec('11011001')  BitMaskRealWorld=Stored Integer
  constant_0 : Constant  Value=0  OutDataTypeStr=fixdt(0, 3, 0)  SampleTime=-1
  constant_1 : Constant  OutDataTypeStr=fixdt(0, 3, 0)  SampleTime=-1
  constant_2 : Constant  Value=2  OutDataTypeStr=fixdt(0, 3, 0)  SampleTime=-1
  delay : Delay  DelayLength=1
  multiport_switch : MultiPortSwitch  DataPortOrder=Zero-based contiguous  zeroidx=on
  rd_address : hdlsllib/Logic and Bit Operations/Bit Slice  lidx=9  ridx=0
      settings: SourceProductName=Simulink  SourceProductBaseCode=SL
  rd_address_hr : hdlsllib/Logic and Bit Operations/Bit Slice  lidx=8  ridx=0
      settings: SourceProductName=Simulink  SourceProductBaseCode=SL
  rd_bitslice : hdlsllib/Logic and Bit Operations/Bit Slice  lidx=11  ridx=10
      settings: SourceProductName=Simulink  SourceProductBaseCode=SL
  rd_cmp2const_0 : simulink/Logic and Bit Operations/Compare To Constant  relop===  const=0  OutDataTypeStr=boolean
  rd_cmp2const_1 : simulink/Logic and Bit Operations/Compare To Constant  relop===  const=1  OutDataTypeStr=boolean
  rd_cmp2const_2 : simulink/Logic and Bit Operations/Compare To Constant  relop===  const=2  OutDataTypeStr=boolean
  simple_ram_0 : hdlsllib/HDL RAMs/Simple Dual Port RAM  ram_size=10
      settings: SourceProductName=Simulink  SourceProductBaseCode=SL
  simple_ram_1 : hdlsllib/HDL RAMs/Simple Dual Port RAM  ram_size=10
      settings: SourceProductName=Simulink  SourceProductBaseCode=SL
  simple_ram_2 : hdlsllib/HDL RAMs/Simple Dual Port RAM  ram_size=9
      settings: SourceProductName=Simulink  SourceProductBaseCode=SL
  switch_0 : Switch  Threshold=1
  switch_1 : Switch  Threshold=1
  switch_2 : Switch  Threshold=1
  vector_concatenate : Concatenate  NumInputs=3
  wr_address : hdlsllib/Logic and Bit Operations/Bit Slice  lidx=9  ridx=0
      settings: SourceProductName=Simulink  SourceProductBaseCode=SL
  wr_address_hr : hdlsllib/Logic and Bit Operations/Bit Slice  lidx=8  ridx=0
      settings: SourceProductName=Simulink  SourceProductBaseCode=SL
  wr_bitslice : hdlsllib/Logic and Bit Operations/Bit Slice  lidx=11  ridx=10
      settings: SourceProductName=Simulink  SourceProductBaseCode=SL
  wr_cmp2const_0 : simulink/Logic and Bit Operations/Compare To Constant  relop===  const=0  OutDataTypeStr=boolean
  wr_cmp2const_1 : simulink/Logic and Bit Operations/Compare To Constant  relop===  const=1  OutDataTypeStr=boolean
  wr_cmp2const_2 : simulink/Logic and Bit Operations/Compare To Constant  relop===  const=2  OutDataTypeStr=boolean
  zero : Constant  Value=0  OutDataTypeStr=fixdt(0, 3, 0)  SampleTime=-1
  rd_data : Outport
  wires:
  rd_addr/1 -> rd_bitslice/1, rd_address_hr/1, rd_address/1
  wr_en/1 -> and_2/2, and_1/2, and_0/2
  wr_addr/1 -> wr_bitslice/1, wr_address_hr/1, wr_address/1
  wr_data/1 -> simple_ram_0/1, simple_ram_1/1, simple_ram_2/1
  and_0/1 -> simple_ram_0/3
  and_1/1 -> simple_ram_1/3
  and_2/1 -> simple_ram_2/3
  bitwise_or/1 -> delay/1
  constant_0/1 -> switch_0/1
  constant_1/1 -> switch_1/1
  constant_2/1 -> switch_2/1
  delay/1 -> multiport_switch/1
  multiport_switch/1 -> rd_data/1
  rd_address/1 -> simple_ram_0/4, simple_ram_1/4
  rd_address_hr/1 -> simple_ram_2/4
  rd_bitslice/1 -> rd_cmp2const_2/1, rd_cmp2const_1/1, rd_cmp2const_0/1
  rd_cmp2const_0/1 -> switch_0/2
  rd_cmp2const_1/1 -> switch_1/2
  rd_cmp2const_2/1 -> switch_2/2
  simple_ram_0/1 -> multiport_switch/2
  simple_ram_1/1 -> multiport_switch/3
  simple_ram_2/1 -> multiport_switch/4
  switch_0/1 -> vector_concatenate/1
  switch_1/1 -> vector_concatenate/2
  switch_2/1 -> vector_concatenate/3
  vector_concatenate/1 -> bitwise_or/1
  wr_address/1 -> simple_ram_0/2, simple_ram_1/2
  wr_address_hr/1 -> simple_ram_2/2
  wr_bitslice/1 -> wr_cmp2const_2/1, wr_cmp2const_1/1, wr_cmp2const_0/1
  wr_cmp2const_0/1 -> and_0/1
  wr_cmp2const_1/1 -> and_1/1
  wr_cmp2const_2/1 -> and_2/1
  zero/1 -> switch_2/3, switch_1/3, switch_0/3

== system gm_hybrid_lht/Hybrid LHT/Hybrid LHT Accumulator/Accumulator with Switches/Accumulator_instance18/Block RAM/Simple Dual Port RAM Generator ==
  wr_data : Inport  OutDataTypeStr=fixdt(0, 36, 0)  PortDimensions=1  SampleTime=8.33333333333333e-09
  wr_addr : Inport  Port=2  OutDataTypeStr=fixdt(0, 12, 0)  PortDimensions=1  SampleTime=8.33333333333333e-09
  wr_en : Inport  Port=3  OutDataTypeStr=boolean  PortDimensions=1  SampleTime=8.33333333333333e-09
  rd_addr : Inport  Port=4  OutDataTypeStr=fixdt(0, 12, 0)  PortDimensions=1  SampleTime=8.33333333333333e-09
  and_0 : Logic  AllPortsSameDT=off  OutDataTypeStr=boolean
  and_1 : Logic  AllPortsSameDT=off  OutDataTypeStr=boolean
  and_2 : Logic  AllPortsSameDT=off  OutDataTypeStr=boolean
  bitwise_or : simulink/Logic and Bit Operations/Bitwise Operator  logicop=OR  UseBitMask=off  BitMask=bin2dec('11011001')  BitMaskRealWorld=Stored Integer
  constant_0 : Constant  Value=0  OutDataTypeStr=fixdt(0, 3, 0)  SampleTime=-1
  constant_1 : Constant  OutDataTypeStr=fixdt(0, 3, 0)  SampleTime=-1
  constant_2 : Constant  Value=2  OutDataTypeStr=fixdt(0, 3, 0)  SampleTime=-1
  delay : Delay  DelayLength=1
  multiport_switch : MultiPortSwitch  DataPortOrder=Zero-based contiguous  zeroidx=on
  rd_address : hdlsllib/Logic and Bit Operations/Bit Slice  lidx=9  ridx=0
      settings: SourceProductName=Simulink  SourceProductBaseCode=SL
  rd_address_hr : hdlsllib/Logic and Bit Operations/Bit Slice  lidx=8  ridx=0
      settings: SourceProductName=Simulink  SourceProductBaseCode=SL
  rd_bitslice : hdlsllib/Logic and Bit Operations/Bit Slice  lidx=11  ridx=10
      settings: SourceProductName=Simulink  SourceProductBaseCode=SL
  rd_cmp2const_0 : simulink/Logic and Bit Operations/Compare To Constant  relop===  const=0  OutDataTypeStr=boolean
  rd_cmp2const_1 : simulink/Logic and Bit Operations/Compare To Constant  relop===  const=1  OutDataTypeStr=boolean
  rd_cmp2const_2 : simulink/Logic and Bit Operations/Compare To Constant  relop===  const=2  OutDataTypeStr=boolean
  simple_ram_0 : hdlsllib/HDL RAMs/Simple Dual Port RAM  ram_size=10
      settings: SourceProductName=Simulink  SourceProductBaseCode=SL
  simple_ram_1 : hdlsllib/HDL RAMs/Simple Dual Port RAM  ram_size=10
      settings: SourceProductName=Simulink  SourceProductBaseCode=SL
  simple_ram_2 : hdlsllib/HDL RAMs/Simple Dual Port RAM  ram_size=9
      settings: SourceProductName=Simulink  SourceProductBaseCode=SL
  switch_0 : Switch  Threshold=1
  switch_1 : Switch  Threshold=1
  switch_2 : Switch  Threshold=1
  vector_concatenate : Concatenate  NumInputs=3
  wr_address : hdlsllib/Logic and Bit Operations/Bit Slice  lidx=9  ridx=0
      settings: SourceProductName=Simulink  SourceProductBaseCode=SL
  wr_address_hr : hdlsllib/Logic and Bit Operations/Bit Slice  lidx=8  ridx=0
      settings: SourceProductName=Simulink  SourceProductBaseCode=SL
  wr_bitslice : hdlsllib/Logic and Bit Operations/Bit Slice  lidx=11  ridx=10
      settings: SourceProductName=Simulink  SourceProductBaseCode=SL
  wr_cmp2const_0 : simulink/Logic and Bit Operations/Compare To Constant  relop===  const=0  OutDataTypeStr=boolean
  wr_cmp2const_1 : simulink/Logic and Bit Operations/Compare To Constant  relop===  const=1  OutDataTypeStr=boolean
  wr_cmp2const_2 : simulink/Logic and Bit Operations/Compare To Constant  relop===  const=2  OutDataTypeStr=boolean
  zero : Constant  Value=0  OutDataTypeStr=fixdt(0, 3, 0)  SampleTime=-1
  rd_data : Outport
  wires:
  rd_addr/1 -> rd_bitslice/1, rd_address_hr/1, rd_address/1
  wr_en/1 -> and_2/2, and_1/2, and_0/2
  wr_addr/1 -> wr_bitslice/1, wr_address_hr/1, wr_address/1
  wr_data/1 -> simple_ram_0/1, simple_ram_1/1, simple_ram_2/1
  and_0/1 -> simple_ram_0/3
  and_1/1 -> simple_ram_1/3
  and_2/1 -> simple_ram_2/3
  bitwise_or/1 -> delay/1
  constant_0/1 -> switch_0/1
  constant_1/1 -> switch_1/1
  constant_2/1 -> switch_2/1
  delay/1 -> multiport_switch/1
  multiport_switch/1 -> rd_data/1
  rd_address/1 -> simple_ram_0/4, simple_ram_1/4
  rd_address_hr/1 -> simple_ram_2/4
  rd_bitslice/1 -> rd_cmp2const_2/1, rd_cmp2const_1/1, rd_cmp2const_0/1
  rd_cmp2const_0/1 -> switch_0/2
  rd_cmp2const_1/1 -> switch_1/2
  rd_cmp2const_2/1 -> switch_2/2
  simple_ram_0/1 -> multiport_switch/2
  simple_ram_1/1 -> multiport_switch/3
  simple_ram_2/1 -> multiport_switch/4
  switch_0/1 -> vector_concatenate/1
  switch_1/1 -> vector_concatenate/2
  switch_2/1 -> vector_concatenate/3
  vector_concatenate/1 -> bitwise_or/1
  wr_address/1 -> simple_ram_0/2, simple_ram_1/2
  wr_address_hr/1 -> simple_ram_2/2
  wr_bitslice/1 -> wr_cmp2const_2/1, wr_cmp2const_1/1, wr_cmp2const_0/1
  wr_cmp2const_0/1 -> and_0/1
  wr_cmp2const_1/1 -> and_1/1
  wr_cmp2const_2/1 -> and_2/1
  zero/1 -> switch_2/3, switch_1/3, switch_0/3

== system gm_hybrid_lht/Hybrid LHT/Hybrid LHT Accumulator/Accumulator with Switches/Accumulator_instance19/Block RAM/Simple Dual Port RAM Generator ==
  wr_data : Inport  OutDataTypeStr=fixdt(0, 36, 0)  PortDimensions=1  SampleTime=8.33333333333333e-09
  wr_addr : Inport  Port=2  OutDataTypeStr=fixdt(0, 12, 0)  PortDimensions=1  SampleTime=8.33333333333333e-09
  wr_en : Inport  Port=3  OutDataTypeStr=boolean  PortDimensions=1  SampleTime=8.33333333333333e-09
  rd_addr : Inport  Port=4  OutDataTypeStr=fixdt(0, 12, 0)  PortDimensions=1  SampleTime=8.33333333333333e-09
  and_0 : Logic  AllPortsSameDT=off  OutDataTypeStr=boolean
  and_1 : Logic  AllPortsSameDT=off  OutDataTypeStr=boolean
  and_2 : Logic  AllPortsSameDT=off  OutDataTypeStr=boolean
  bitwise_or : simulink/Logic and Bit Operations/Bitwise Operator  logicop=OR  UseBitMask=off  BitMask=bin2dec('11011001')  BitMaskRealWorld=Stored Integer
  constant_0 : Constant  Value=0  OutDataTypeStr=fixdt(0, 3, 0)  SampleTime=-1
  constant_1 : Constant  OutDataTypeStr=fixdt(0, 3, 0)  SampleTime=-1
  constant_2 : Constant  Value=2  OutDataTypeStr=fixdt(0, 3, 0)  SampleTime=-1
  delay : Delay  DelayLength=1
  multiport_switch : MultiPortSwitch  DataPortOrder=Zero-based contiguous  zeroidx=on
  rd_address : hdlsllib/Logic and Bit Operations/Bit Slice  lidx=9  ridx=0
      settings: SourceProductName=Simulink  SourceProductBaseCode=SL
  rd_address_hr : hdlsllib/Logic and Bit Operations/Bit Slice  lidx=8  ridx=0
      settings: SourceProductName=Simulink  SourceProductBaseCode=SL
  rd_bitslice : hdlsllib/Logic and Bit Operations/Bit Slice  lidx=11  ridx=10
      settings: SourceProductName=Simulink  SourceProductBaseCode=SL
  rd_cmp2const_0 : simulink/Logic and Bit Operations/Compare To Constant  relop===  const=0  OutDataTypeStr=boolean
  rd_cmp2const_1 : simulink/Logic and Bit Operations/Compare To Constant  relop===  const=1  OutDataTypeStr=boolean
  rd_cmp2const_2 : simulink/Logic and Bit Operations/Compare To Constant  relop===  const=2  OutDataTypeStr=boolean
  simple_ram_0 : hdlsllib/HDL RAMs/Simple Dual Port RAM  ram_size=10
      settings: SourceProductName=Simulink  SourceProductBaseCode=SL
  simple_ram_1 : hdlsllib/HDL RAMs/Simple Dual Port RAM  ram_size=10
      settings: SourceProductName=Simulink  SourceProductBaseCode=SL
  simple_ram_2 : hdlsllib/HDL RAMs/Simple Dual Port RAM  ram_size=9
      settings: SourceProductName=Simulink  SourceProductBaseCode=SL
  switch_0 : Switch  Threshold=1
  switch_1 : Switch  Threshold=1
  switch_2 : Switch  Threshold=1
  vector_concatenate : Concatenate  NumInputs=3
  wr_address : hdlsllib/Logic and Bit Operations/Bit Slice  lidx=9  ridx=0
      settings: SourceProductName=Simulink  SourceProductBaseCode=SL
  wr_address_hr : hdlsllib/Logic and Bit Operations/Bit Slice  lidx=8  ridx=0
      settings: SourceProductName=Simulink  SourceProductBaseCode=SL
  wr_bitslice : hdlsllib/Logic and Bit Operations/Bit Slice  lidx=11  ridx=10
      settings: SourceProductName=Simulink  SourceProductBaseCode=SL
  wr_cmp2const_0 : simulink/Logic and Bit Operations/Compare To Constant  relop===  const=0  OutDataTypeStr=boolean
  wr_cmp2const_1 : simulink/Logic and Bit Operations/Compare To Constant  relop===  const=1  OutDataTypeStr=boolean
  wr_cmp2const_2 : simulink/Logic and Bit Operations/Compare To Constant  relop===  const=2  OutDataTypeStr=boolean
  zero : Constant  Value=0  OutDataTypeStr=fixdt(0, 3, 0)  SampleTime=-1
  rd_data : Outport
  wires:
  rd_addr/1 -> rd_bitslice/1, rd_address_hr/1, rd_address/1
  wr_en/1 -> and_2/2, and_1/2, and_0/2
  wr_addr/1 -> wr_bitslice/1, wr_address_hr/1, wr_address/1
  wr_data/1 -> simple_ram_0/1, simple_ram_1/1, simple_ram_2/1
  and_0/1 -> simple_ram_0/3
  and_1/1 -> simple_ram_1/3
  and_2/1 -> simple_ram_2/3
  bitwise_or/1 -> delay/1
  constant_0/1 -> switch_0/1
  constant_1/1 -> switch_1/1
  constant_2/1 -> switch_2/1
  delay/1 -> multiport_switch/1
  multiport_switch/1 -> rd_data/1
  rd_address/1 -> simple_ram_0/4, simple_ram_1/4
  rd_address_hr/1 -> simple_ram_2/4
  rd_bitslice/1 -> rd_cmp2const_2/1, rd_cmp2const_1/1, rd_cmp2const_0/1
  rd_cmp2const_0/1 -> switch_0/2
  rd_cmp2const_1/1 -> switch_1/2
  rd_cmp2const_2/1 -> switch_2/2
  simple_ram_0/1 -> multiport_switch/2
  simple_ram_1/1 -> multiport_switch/3
  simple_ram_2/1 -> multiport_switch/4
  switch_0/1 -> vector_concatenate/1
  switch_1/1 -> vector_concatenate/2
  switch_2/1 -> vector_concatenate/3
  vector_concatenate/1 -> bitwise_or/1
  wr_address/1 -> simple_ram_0/2, simple_ram_1/2
  wr_address_hr/1 -> simple_ram_2/2
  wr_bitslice/1 -> wr_cmp2const_2/1, wr_cmp2const_1/1, wr_cmp2const_0/1
  wr_cmp2const_0/1 -> and_0/1
  wr_cmp2const_1/1 -> and_1/1
  wr_cmp2const_2/1 -> and_2/1
  zero/1 -> switch_2/3, switch_1/3, switch_0/3

== system gm_hybrid_lht/Hybrid LHT/Hybrid LHT Accumulator/Accumulator with Switches/Accumulator_instance2/Block RAM/Simple Dual Port RAM Generator ==
  wr_data : Inport  OutDataTypeStr=fixdt(0, 36, 0)  PortDimensions=1  SampleTime=8.33333333333333e-09
  wr_addr : Inport  Port=2  OutDataTypeStr=fixdt(0, 12, 0)  PortDimensions=1  SampleTime=8.33333333333333e-09
  wr_en : Inport  Port=3  OutDataTypeStr=boolean  PortDimensions=1  SampleTime=8.33333333333333e-09
  rd_addr : Inport  Port=4  OutDataTypeStr=fixdt(0, 12, 0)  PortDimensions=1  SampleTime=8.33333333333333e-09
  and_0 : Logic  AllPortsSameDT=off  OutDataTypeStr=boolean
  and_1 : Logic  AllPortsSameDT=off  OutDataTypeStr=boolean
  and_2 : Logic  AllPortsSameDT=off  OutDataTypeStr=boolean
  bitwise_or : simulink/Logic and Bit Operations/Bitwise Operator  logicop=OR  UseBitMask=off  BitMask=bin2dec('11011001')  BitMaskRealWorld=Stored Integer
  constant_0 : Constant  Value=0  OutDataTypeStr=fixdt(0, 3, 0)  SampleTime=-1
  constant_1 : Constant  OutDataTypeStr=fixdt(0, 3, 0)  SampleTime=-1
  constant_2 : Constant  Value=2  OutDataTypeStr=fixdt(0, 3, 0)  SampleTime=-1
  delay : Delay  DelayLength=1
  multiport_switch : MultiPortSwitch  DataPortOrder=Zero-based contiguous  zeroidx=on
  rd_address : hdlsllib/Logic and Bit Operations/Bit Slice  lidx=9  ridx=0
      settings: SourceProductName=Simulink  SourceProductBaseCode=SL
  rd_address_hr : hdlsllib/Logic and Bit Operations/Bit Slice  lidx=8  ridx=0
      settings: SourceProductName=Simulink  SourceProductBaseCode=SL
  rd_bitslice : hdlsllib/Logic and Bit Operations/Bit Slice  lidx=11  ridx=10
      settings: SourceProductName=Simulink  SourceProductBaseCode=SL
  rd_cmp2const_0 : simulink/Logic and Bit Operations/Compare To Constant  relop===  const=0  OutDataTypeStr=boolean
  rd_cmp2const_1 : simulink/Logic and Bit Operations/Compare To Constant  relop===  const=1  OutDataTypeStr=boolean
  rd_cmp2const_2 : simulink/Logic and Bit Operations/Compare To Constant  relop===  const=2  OutDataTypeStr=boolean
  simple_ram_0 : hdlsllib/HDL RAMs/Simple Dual Port RAM  ram_size=10
      settings: SourceProductName=Simulink  SourceProductBaseCode=SL
  simple_ram_1 : hdlsllib/HDL RAMs/Simple Dual Port RAM  ram_size=10
      settings: SourceProductName=Simulink  SourceProductBaseCode=SL
  simple_ram_2 : hdlsllib/HDL RAMs/Simple Dual Port RAM  ram_size=9
      settings: SourceProductName=Simulink  SourceProductBaseCode=SL
  switch_0 : Switch  Threshold=1
  switch_1 : Switch  Threshold=1
  switch_2 : Switch  Threshold=1
  vector_concatenate : Concatenate  NumInputs=3
  wr_address : hdlsllib/Logic and Bit Operations/Bit Slice  lidx=9  ridx=0
      settings: SourceProductName=Simulink  SourceProductBaseCode=SL
  wr_address_hr : hdlsllib/Logic and Bit Operations/Bit Slice  lidx=8  ridx=0
      settings: SourceProductName=Simulink  SourceProductBaseCode=SL
  wr_bitslice : hdlsllib/Logic and Bit Operations/Bit Slice  lidx=11  ridx=10
      settings: SourceProductName=Simulink  SourceProductBaseCode=SL
  wr_cmp2const_0 : simulink/Logic and Bit Operations/Compare To Constant  relop===  const=0  OutDataTypeStr=boolean
  wr_cmp2const_1 : simulink/Logic and Bit Operations/Compare To Constant  relop===  const=1  OutDataTypeStr=boolean
  wr_cmp2const_2 : simulink/Logic and Bit Operations/Compare To Constant  relop===  const=2  OutDataTypeStr=boolean
  zero : Constant  Value=0  OutDataTypeStr=fixdt(0, 3, 0)  SampleTime=-1
  rd_data : Outport
  wires:
  rd_addr/1 -> rd_bitslice/1, rd_address_hr/1, rd_address/1
  wr_en/1 -> and_2/2, and_1/2, and_0/2
  wr_addr/1 -> wr_bitslice/1, wr_address_hr/1, wr_address/1
  wr_data/1 -> simple_ram_0/1, simple_ram_1/1, simple_ram_2/1
  and_0/1 -> simple_ram_0/3
  and_1/1 -> simple_ram_1/3
  and_2/1 -> simple_ram_2/3
  bitwise_or/1 -> delay/1
  constant_0/1 -> switch_0/1
  constant_1/1 -> switch_1/1
  constant_2/1 -> switch_2/1
  delay/1 -> multiport_switch/1
  multiport_switch/1 -> rd_data/1
  rd_address/1 -> simple_ram_0/4, simple_ram_1/4
  rd_address_hr/1 -> simple_ram_2/4
  rd_bitslice/1 -> rd_cmp2const_2/1, rd_cmp2const_1/1, rd_cmp2const_0/1
  rd_cmp2const_0/1 -> switch_0/2
  rd_cmp2const_1/1 -> switch_1/2
  rd_cmp2const_2/1 -> switch_2/2
  simple_ram_0/1 -> multiport_switch/2
  simple_ram_1/1 -> multiport_switch/3
  simple_ram_2/1 -> multiport_switch/4
  switch_0/1 -> vector_concatenate/1
  switch_1/1 -> vector_concatenate/2
  switch_2/1 -> vector_concatenate/3
  vector_concatenate/1 -> bitwise_or/1
  wr_address/1 -> simple_ram_0/2, simple_ram_1/2
  wr_address_hr/1 -> simple_ram_2/2
  wr_bitslice/1 -> wr_cmp2const_2/1, wr_cmp2const_1/1, wr_cmp2const_0/1
  wr_cmp2const_0/1 -> and_0/1
  wr_cmp2const_1/1 -> and_1/1
  wr_cmp2const_2/1 -> and_2/1
  zero/1 -> switch_2/3, switch_1/3, switch_0/3
